simulink model "ECOS"  (R2025a)
settings: Solver=VariableStepAuto  StartTime=0.0  StopTime=1  RelTol=1e-3
settings Model: Creator=JR  LastModifiedBy=JR

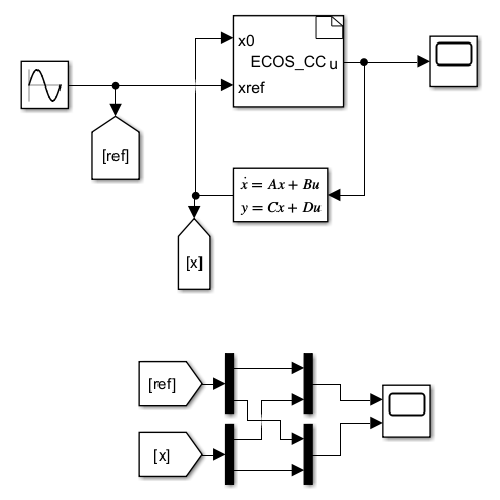
[thumbnail: Simulink's stored preview of the top-level diagram]
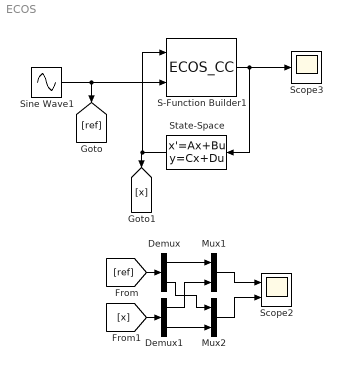
== system ECOS ==
  Demux : Demux  Outputs=2
  Demux1 : Demux  Outputs=2
  Mux1 : Mux  Inputs=2
  Mux2 : Mux  Inputs=2
  S-Function Builder1 : S-Function  FunctionName=ECOS_CC  SFunctionModules=ECOS_CC_wrapper.c cpg_workspace cpg_solve cone ctrlc ecos equil kkt preproc spla splamm timer wright_omega ldl amd_1 amd_2 amd_aat amd_control amd_defaults amd_dump amd_global amd_info amd_order amd_post_tree amd_postorder amd_preprocess amd_valid ecos_bb ecos_bb_preproc expcone  SFunctionDeploymentMode=off  EnableBusSupport=off  mask(S-Function Builder){}
      mask help: Simulink:masks:SFunctionBuilder_MD
      mask init:
      | val = [[.9  0.75 0.75 1 1 .9 .9 1]',[1 1 0.75 0.75 .9 .9 1 .9]'];try , sys = get_param(gcb,'SfunBuilderFcnName');if isempty(sys), sys = get_param(gcb,'FunctionName'); end,catch, sys = get_param(gcb,'FunctionName'); end
      settings: CopyFcn=set_param(gcbh,'LinkStatus','none')  OpenFcn=sfunctionwizard(gcbh)
      mask Display:
      | plot(val(:,1),val(:,2))
      | disp(sys)
      | port_label('input',1,sprintf('%s', 'x0'),'interpreter','tex')
      | port_label('input',2,sprintf('%s', 'xref'),'interpreter','tex')
      | port_label('output',1,sprintf('%s', 'u'),'interpreter','tex')
  Scope2 : Scope  NumInputPorts=2
      settings: ActiveDisplayYMinimum=-2.4999999680253175  ActiveDisplayYMaximum=2.4999999964472575  DataLoggingVariableName=ScopeData2
  Scope3 : Scope
      settings: ActiveDisplayYMinimum=-59.152382824378776  ActiveDisplayYMaximum=74.177997372903562  DataLoggingVariableName=ScopeData3
  Sine Wave1 : Sin  Amplitude=[1;1]  Frequency=100  Phase=[0;pi/2]  SampleTime=0
  State-Space : StateSpace  A=[0 0;0 0]  B=[-400 0; 0 -400]  C=[1 0;0 1]  D=[0 0;0 0]  InitialCondition=[2 ;-1]
  wires:
  Demux/1 -> Mux1/1
  Demux/2 -> Mux2/1
  State-Space/1 -> S-Function Builder1/1, [x]
  Mux2/1 -> Scope2/2
  Demux1/2 -> Mux2/2
  S-Function Builder1/1 -> State-Space/1, Scope3/1
  [x] -> Demux1/1
  [ref] -> Demux/1
  Sine Wave1/1 -> S-Function Builder1/2, [ref]
  Mux1/1 -> Scope2/1
  Demux1/1 -> Mux1/2
